simulink model "agentsim"  (R2018b)
settings: Solver=ode4  StartTime=0.0  StopTime=1  FixedStep=0.001  RelTol=1e-3  EnableMultiTasking=on
settings Model: ExtModeTrigMode=oneshot  ExtModeArmWhenConnect=off  Creator=hp  LastModifiedBy=Administrator
settings DataIOCC: SaveFormat=Array  SignalLoggingSaveFormat=ModelDataLogs  SignalLoggingName=sigsOut
settings OptimizationCC: BooleanDataType=off  ExpressionDepthLimit=2147483647  InitFltsAndDblsToZero=on  LifeSpan=inf
settings DebuggingCC: SaveWithParameterizedLinksMsg=none  UnderspecifiedInitializationDetection=Classic  MergeDetectMultiDrivingBlocksExec=none  SignalResolutionControl=TryResolveAllWithWarning  MultiTaskDSMMsg=warning  MultiTaskCondExecSysMsg=none  FcnCallInpInsideContextMsg=warning  StateNameClashWarn=warning  SFUnexpectedBacktrackingDiag=warning  SFNoUnconditionalDefaultTransitionDiag=warning  SFExecutionAtInitializationDiag=none
settings HardwareCC: ProdBitPerPointer=32  ProdBitPerSizeT=32  ProdBitPerPtrDiffT=32  ProdLargestAtomicFloat=None  ProdIntDivRoundTo=Undefined  ProdEndianess=Unspecified  ProdWordSize=32  ProdHWDeviceType=32-bit Generic  TargetUnknown=on
settings ModelReferenceCC: PropagateSignalLabelsOutOfModel=off
settings SFSimCC: SimUseLocalCustomCode=off
settings RTWCC: RTWUseLocalCustomCode=off
settings CodeAppCC: StateflowObjectComments=on
settings GRTTargetCC: TargetFcnLib=ansi_tfl_tmw.mat  TargetLangStandard=C89/C90 (ANSI)  GeneratePreprocessorConditionals=Disable all  CombineOutputUpdateFcns=off  GRTInterface=on
settings ConfigComp: CovMetricSettings=dw  CovHtmlReporting=on  CovSaveCumulativeToWorkspaceVar=on  CovSaveSingleToWorkspaceVar=on  CovExternalEMLEnable=off

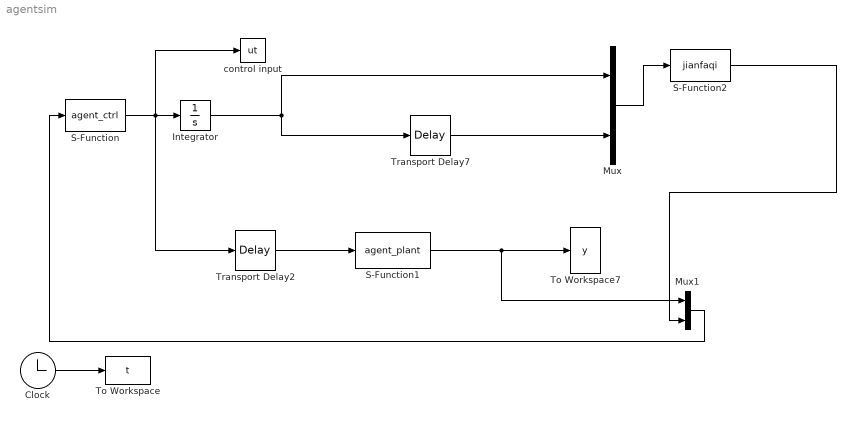
== system agentsim ==
  Clock : Clock
  Integrator : Integrator
  Mux : Mux  Inputs=2
  Mux1 : Mux  Inputs=2
  S-Function : S-Function  FunctionName=agent_ctrl  SFunctionDeploymentMode=off  EnableBusSupport=off
  S-Function1 : S-Function  FunctionName=agent_plant  SFunctionDeploymentMode=off  EnableBusSupport=off
  S-Function2 : S-Function  FunctionName=jianfaqi  SFunctionDeploymentMode=off  EnableBusSupport=off
  To Workspace : ToWorkspace  VariableName=t  SampleTime=-1
  To Workspace7 : ToWorkspace  VariableName=y  SampleTime=-1
  Transport Delay2 : TransportDelay  DelayTime=0.06
  Transport Delay7 : TransportDelay  DelayTime=0.06
  control input : ToWorkspace  VariableName=ut  SampleTime=-1
  wires:
  Clock/1 -> To Workspace/1
  S-Function1/1 -> Mux1/1, To Workspace7/1
  S-Function/1 -> Transport Delay2/1, control input/1, Integrator/1
  Mux/1 -> S-Function2/1
  S-Function2/1 -> Mux1/2
  Mux1/1 -> S-Function/1
  Transport Delay2/1 -> S-Function1/1
  Integrator/1 -> Mux/1, Transport Delay7/1
  Transport Delay7/1 -> Mux/2
